simulink model "mesure_freq"  (R2022b)
settings: Solver=VariableStepAuto  StartTime=0.0  StopTime=10.0  RelTol=1e-3
settings Model: Creator=antoine  LastModifiedBy=antoine

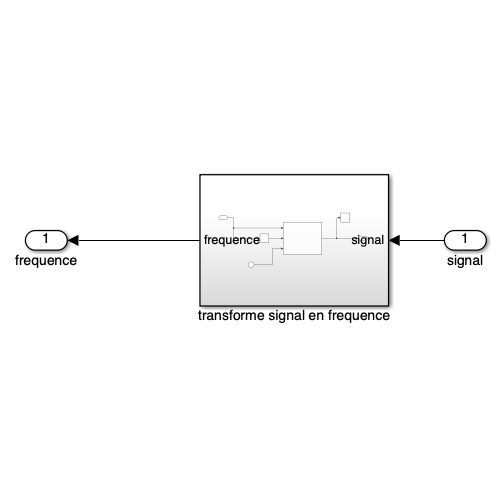
[thumbnail: Simulink's stored preview of the top-level diagram]
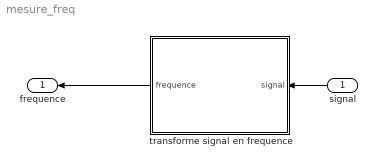
== system mesure_freq ==
  signal : Inport
  transforme signal en frequence : Subsystem
  frequence : Outport
  wires:
  transforme signal en frequence/1(frequence) -> frequence/1
  signal/1 -> transforme signal en frequence/1(signal)

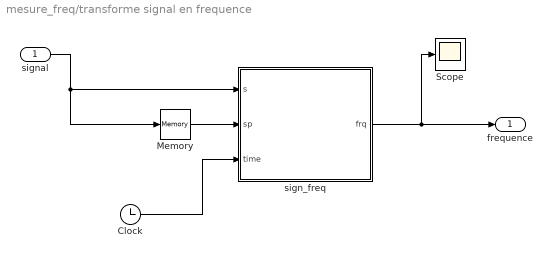
== system mesure_freq/transforme signal en frequence ==
  signal : Inport
  Clock : Clock
  Memory : Memory
  Scope : Scope
  sign_freq : MATLAB Function  TreatAsAtomicUnit=on
  frequence : Outport
  wires:
  signal/1 -> Memory/1, sign_freq/1(s)
  sign_freq/1(frq) -> Scope/1, frequence/1
  Clock/1 -> sign_freq/3(time)
  Memory/1 -> sign_freq/2(sp)

== matlab function mesure_freq/transforme signal en frequence/sign_freq ==
  settings: updateMethod=DISCRETE
  data: s input; sp input; frq output; time input
function frq = sign_freq(s, sp, time)
persistent up_timer;
persistent down_timer;
% section pour pas avoir de bug
if isempty(up_timer)
    up_timer = 0;
end
if isempty(down_timer)
    down_timer = 0;
    frq = 100;
end
% pas de bug



if s == 5 && sp ~= 5 % debut du up
    up_timer = time;
elseif s == 0 && sp ~= 0 % debut du down
    down_timer = time;
end
period = abs((up_timer-down_timer)*2);
frq = 1/period;
